simulink model "MIL4L3_SW6_V1_20220211"  (R2018b)
settings: Solver=FixedStepAuto  StartTime=0.0  StopTime=inf  FixedStep=0.001  RelTol=1e-3
PreLoadFcn:
  | A0_MILtest;
undefined symbols (not defined in the file or in its folder): Clb_ICADirect_LaneDisp_StateFive, Clb_ICADirect_LaneDisp_StateFour, Clb_ICADirect_LaneDisp_StateOne, Clb_ICADirect_LaneDisp_StateThree, Clb_ICADirect_LaneDisp_StateTwo, Clb_ICADirect_LaneDisp_StateZero, Clb_ICADirect_LaneDispSW, Clb_ICADirect_TrnLghtsCom_Switch, Clb_ICADirect_TrnLghtsCom_Value, Clb_ICADirect_TrnLghtsCrtl_Inhb, IMAP_Clb_ACU_Driver_Belt, IMAP_Clb_ACU_Driver_Belt_Over, IMAP_Clb_ACU_Passenger_Belt, IMAP_Clb_ACU_Passenger_Belt_Over, IMAP_Clb_ACU_RearLeft_Belt, IMAP_Clb_ACU_RearLeft_Belt_Over, IMAP_Clb_ACU_RearMiddle_Belt, IMAP_Clb_ACU_RearMiddle_Belt_Over, IMAP_Clb_ACU_RearRight_Belt, IMAP_Clb_ACU_RearRight_Belt_Over, IMAP_Clb_AEB_Switch, IMAP_Clb_AEB_Switch_Over, IMAP_Clb_ALC_TLC_Mode, IMAP_Clb_ALC_TLC_Mode_Over, IMAP_Clb_BCM_Battery_Voltage, IMAP_Clb_BCM_Battery_Voltage_Over, IMAP_Clb_BCM_BrakeLamp_State, IMAP_Clb_BCM_BrakeLamp_State_Over, IMAP_Clb_BCM_CHMSL_Status, IMAP_Clb_BCM_CHMSL_Status_Over, IMAP_Clb_BCM_Door_Lock_State, IMAP_Clb_BCM_Door_Lock_State_Over, IMAP_Clb_BCM_FrontWiper_State, IMAP_Clb_BCM_FrontWiper_State_Over, IMAP_Clb_BCM_FrontWiper_Switch, IMAP_Clb_BCM_FrontWiper_Switch_Over, IMAP_Clb_BCM_HazardLamp, IMAP_Clb_BCM_HazardLamp_Over, IMAP_Clb_BCM_HazardLamp_Switch, IMAP_Clb_BCM_HazardLamp_Switch_Over, IMAP_Clb_BCM_HighBeam_State, IMAP_Clb_BCM_HighBeam_State_Over, IMAP_Clb_BCM_Ignition_State, IMAP_Clb_BCM_Ignition_State_Over, IMAP_Clb_BCM_IHBC_Enabled, IMAP_Clb_BCM_IHBC_Enabled_Over, IMAP_Clb_BCM_Left_Light, IMAP_Clb_BCM_Left_Light_Over, IMAP_Clb_BCM_LeftTurn_Switch, IMAP_Clb_BCM_LeftTurn_Switch_Over, IMAP_Clb_BCM_LF_Door_State, IMAP_Clb_BCM_LF_Door_State_Over, IMAP_Clb_BCM_LowBeam_State, IMAP_Clb_BCM_LowBeam_State_Over, IMAP_Clb_BCM_LR_Door_State, IMAP_Clb_BCM_LR_Door_State_Over, IMAP_Clb_BCM_RF_Door_State, IMAP_Clb_BCM_RF_Door_State_Over, IMAP_Clb_BCM_Right_Light, IMAP_Clb_BCM_Right_Light_Over ... (+547)
libraries: CarMaker4SL x2153, simulink x292, dspstat3 x3, canmsglib x2, simulink_extras x1
(part 50 of 52)

== system MIL4L3_SW6_V1_20220211/CarMaker/VehicleControl/OMAP/OMAP1/Runnable_OMAP_10ms_sys/OMAP_Module/ICA_Direct_G59/ICA_Define/Subsystem1/Dspl/DsplPrcs/Txt/TxtFromACC ==
  note: 有没有收到方向盘限幅的影响
  note: 用于放弃变道的接管预留
  TxtFromACC_stTHState : Inport
  TxtFromACC_stLstTHState : Inport  Port=2
  TxtFromACC_stACCTxtDspl : Inport  Port=3
  TxtFromACC_stSWALimFlg : Inport  Port=4
  TxtFromACC_tiSWALimFlgDetnum : Inport  Port=5
  TxtFromACC_stTkOvStChk : Inport  Port=6
  TxtFromACC_tfAddVocCmd : Inport  Port=7
  TxtFromACC_stVehSty : Inport  Port=8
  Compare To Constant : simulink/Logic and Bit Operations/Compare To Constant  relop===  const=uint16(3)  OutDataTypeStr=boolean
  Compare To Zero : simulink/Logic and Bit Operations/Compare To Zero  relop===  OutDataTypeStr=boolean
  Constant{1,3,5,7,9,11,13,15,17,19} (10 alike) : Constant  OutDataTypeStr=uint16
  Constant{2,4,6,8,10,12,14,16,18,20} (10 alike) : Constant  Value=0  OutDataTypeStr=uint16
  Data Type Conversion14 : DataTypeConversion  OutDataTypeStr=uint16
  Data Type Conversion2 : DataTypeConversion  OutDataTypeStr=uint16
  Enabled Subsystem : Subsystem  TreatAsAtomicUnit=on
  Hold : Subsystem  TreatAsAtomicUnit=on
  If : If  NumInputs=2  IfExpression=( u1 == 3 |u1 == 4 |u1 == 6 )& u2 == 6
  If1 : If  NumInputs=2  IfExpression=( u1 == 3 |u1 == 4 |u1 == 6 )& u2 == 7
  If2 : If  NumInputs=2  IfExpression=( u1 == 3 |u1 == 4 |u1 == 6 )& u2 == 8
  If3 : If  NumInputs=3  IfExpression=u1 == 5 & u2 == 2 & u3 == 0
  If4 : If  NumInputs=2  IfExpression=u1 == 1  ElseIfExpressions=u2 == 1
  If5 : If  NumInputs=2  IfExpression=( u1 == 3 |u1 == 4 |u1 == 6 )& u2 == 12
  If6 : If  NumInputs=2  IfExpression=( u1 == 3 |u1 == 4 |u1 == 6 )& u2 == 13
  If7 : If  NumInputs=2  IfExpression=( u1 == 3 |u1 == 4 |u1 == 6 )& u2 == 14
  If8 : If  NumInputs=2  IfExpression=( u1 == 3 |u1 == 4 )& u2 == 15
  If9 : If  NumInputs=2  IfExpression=( u1 == 3 |u1 == 4 )& u2 == 16
  Logical Operator : Logic  Operator=OR  AllPortsSameDT=off  OutDataTypeStr=boolean
  Logical Operator1 : Logic  Inputs=3  AllPortsSameDT=off  OutDataTypeStr=boolean
  Logical Operator2 : Logic  Operator=OR  AllPortsSameDT=off  OutDataTypeStr=boolean
  Merge{,1..3,5..9} (9 alike) : Merge
  Merge4 : Merge  Inputs=3
  RdrBlkInhib : Subsystem
  Start : Subsystem  TreatAsAtomicUnit=on
  Start1 : Subsystem  TreatAsAtomicUnit=on
  Start2 : Subsystem  TreatAsAtomicUnit=on
  Start3 : Subsystem  TreatAsAtomicUnit=on
  Start4 : Subsystem  TreatAsAtomicUnit=on
  Start5 : Subsystem  TreatAsAtomicUnit=on
  Start6 : Subsystem  TreatAsAtomicUnit=on
  Start7 : Subsystem  TreatAsAtomicUnit=on
  Start8 : Subsystem  TreatAsAtomicUnit=on
  Start9 : Subsystem  TreatAsAtomicUnit=on
  Stop : Subsystem  TreatAsAtomicUnit=on
  Stop1 : Subsystem  TreatAsAtomicUnit=on
  Stop2 : Subsystem  TreatAsAtomicUnit=on
  Stop3 : Subsystem  TreatAsAtomicUnit=on
  Stop4 : Subsystem  TreatAsAtomicUnit=on
  Stop5 : Subsystem  TreatAsAtomicUnit=on
  Stop6 : Subsystem  TreatAsAtomicUnit=on
  Stop7 : Subsystem  TreatAsAtomicUnit=on
  Stop8 : Subsystem  TreatAsAtomicUnit=on
  Stop9 : Subsystem  TreatAsAtomicUnit=on
  Unit Delay1 : UnitDelay  SampleTime=-1
  TxtFromACC_stGoReq : Outport
  TxtFromACC_stTkOv : Outport  Port=2
  TxtFromACC_stImmdTkOv : Outport  Port=3
  TxtFromACC_stRdrBlk : Outport  Port=4
  TxtFromACC_stPressSet : Outport  Port=5
  TxtFromACC_stResEPB : Outport  Port=6
  TxtFromACC_stResBrkPedal : Outport  Port=7
  TxtFromACC_stISAToOn : Outport  Port=8
  TxtFromACC_stISAToOff : Outport  Port=9
  wires:
  Stop/1(Out1) -> Merge/2
  Constant2/1 -> Stop/1(In1)
  If/1 -> Start/Action
  Constant1/1 -> Start/1(In1)
  Start/1(Out1) -> Merge/1
  Merge/1 -> TxtFromACC_stGoReq/1
  If/2 -> Stop/Action
  TxtFromACC_stTHState/1 -> [THState]
  If1/2 -> Stop1/Action
  Stop1/1(Out1) -> Merge1/2
  Start1/1(Out1) -> Merge1/1
  Constant4/1 -> Stop1/1(In1)
  If1/1 -> Start1/Action
  Merge1/1 -> TxtFromACC_stTkOv/1
  Constant3/1 -> Start1/1(In1)
  If2/2 -> Stop2/Action
  Stop2/1(Out1) -> Merge2/2
  Start2/1(Out1) -> Merge2/1
  Constant6/1 -> Stop2/1(In1)
  If2/1 -> Start2/Action
  Constant5/1 -> Start2/1(In1)
  TxtFromACC_stLstTHState/1 -> RdrBlkInhib/2(RdrBlkInhib_stLstTHState)
  TxtFromACC_stACCTxtDspl/1 -> [ACCTxtDspl]
  [THState] -> If/1
  [ACCTxtDspl] -> If/2
  [THState] -> If1/1
  [ACCTxtDspl] -> If1/2
  [THState] -> If2/1
  [ACCTxtDspl] -> If2/2
  [THState] -> RdrBlkInhib/1(RdrBlkInhib_stTHState)
  [ACCTxtDspl] -> RdrBlkInhib/3(RdrBlkInhib_stACCTxtDspl)
  If3/2 -> Stop3/Action
  Start3/1(Out1) -> Merge3/1
  If3/1 -> Start3/Action
  Constant7/1 -> Start3/1(In1)
  Constant8/1 -> Stop3/1(In1)
  Stop3/1(Out1) -> Merge3/2
  [ACCTxtDspl] -> If3/2
  [THState] -> If3/1
  Merge3/1 -> TxtFromACC_stRdrBlk/1
  RdrBlkInhib/1(RdrBlkInhib_stRdrBlkInhibFlg) -> If3/3
  TxtFromACC_stSWALimFlg/1 -> Logical Operator1/3
  TxtFromACC_stTkOvStChk/1 -> If4/2
  If4/2 -> Stop4/Action
  Stop4/1(Out1) -> Merge4/2
  Start4/1(Out1) -> Merge4/1
  Constant10/1 -> Stop4/1(In1)
  If4/1 -> Start4/Action
  Constant9/1 -> Start4/1(In1)
  Hold/1(Out1) -> Merge4/3
  Unit Delay1/1 -> Hold/1(In1)
  Merge4/1 -> Logical Operator/2, Unit Delay1/1
  If4/3 -> Hold/Action
  Merge2/1 -> Logical Operator/1
  Logical Operator/1 -> Data Type Conversion14/1
  Data Type Conversion14/1 -> TxtFromACC_stImmdTkOv/1
  [THState] -> Compare To Constant/1
  Compare To Constant/1 -> Logical Operator1/2
  Data Type Conversion2/1 -> If4/1
  TxtFromACC_tiSWALimFlgDetnum/1 -> Enabled Subsystem/1(Num)
  Enabled Subsystem/1(Triger) -> Logical Operator2/1
  Logical Operator1/1 -> Enabled Subsystem/Enable
  [ACCTxtDspl] -> If5/2
  [THState] -> If5/1
  If5/2 -> Stop5/Action
  Merge5/1 -> TxtFromACC_stPressSet/1
  Start5/1(Out1) -> Merge5/1
  Constant11/1 -> Start5/1(In1)
  If5/1 -> Start5/Action
  Constant12/1 -> Stop5/1(In1)
  Stop5/1(Out1) -> Merge5/2
  Stop6/1(Out1) -> Merge6/2
  Constant14/1 -> Stop6/1(In1)
  If6/1 -> Start6/Action
  Constant13/1 -> Start6/1(In1)
  Start6/1(Out1) -> Merge6/1
  Merge6/1 -> TxtFromACC_stResEPB/1
  If6/2 -> Stop6/Action
  [THState] -> If6/1
  [ACCTxtDspl] -> If6/2
  [ACCTxtDspl] -> If7/2
  [THState] -> If7/1
  If7/2 -> Stop7/Action
  Merge7/1 -> TxtFromACC_stResBrkPedal/1
  Start7/1(Out1) -> Merge7/1
  Constant15/1 -> Start7/1(In1)
  If7/1 -> Start7/Action
  Constant16/1 -> Stop7/1(In1)
  Stop7/1(Out1) -> Merge7/2
  Stop8/1(Out1) -> Merge8/2
  Constant18/1 -> Stop8/1(In1)
  If8/1 -> Start8/Action
  Constant17/1 -> Start8/1(In1)
  Start8/1(Out1) -> Merge8/1
  Merge8/1 -> TxtFromACC_stISAToOn/1
  If8/2 -> Stop8/Action
  [THState] -> If8/1
  [ACCTxtDspl] -> If8/2
  [ACCTxtDspl] -> If9/2
  [THState] -> If9/1
  If9/2 -> Stop9/Action
  Merge9/1 -> TxtFromACC_stISAToOff/1
  Start9/1(Out1) -> Merge9/1
  Constant19/1 -> Start9/1(In1)
  If9/1 -> Start9/Action
  Constant20/1 -> Stop9/1(In1)
  Stop9/1(Out1) -> Merge9/2
  TxtFromACC_tfAddVocCmd/1 -> Logical Operator2/2
  Logical Operator2/1 -> Data Type Conversion2/1
  Compare To Zero/1 -> Logical Operator1/1
  TxtFromACC_stVehSty/1 -> Compare To Zero/1

== system MIL4L3_SW6_V1_20220211/CarMaker/VehicleControl/OMAP/OMAP1/Runnable_OMAP_10ms_sys/OMAP_Module/ICA_Direct_G59/ICA_Define/Subsystem1/Dspl/DsplPrcs/Txt/TxtInactv ==
  TxtInactv_stTHState : Inport
  TxtInactv_stTHFKeyState : Inport  Port=2
  TxtInactv_stCntRst : Inport  Port=3
  Constant1 : Constant  OutDataTypeStr=uint16
  Constant2 : Constant  Value=0  OutDataTypeStr=uint16
  Hold : Subsystem  TreatAsAtomicUnit=on
  If : If  NumInputs=3  IfExpression=u1 ~= 1 | u3 == 1  ElseIfExpressions=u1 == 1 & (u2 == 3 | u2 == 4)
  Merge : Merge  Inputs=3
  Start : Subsystem  TreatAsAtomicUnit=on
  Stop : Subsystem  TreatAsAtomicUnit=on
  Unit Delay1 : UnitDelay  SampleTime=-1
  TxtInactv_stInactv : Outport
  wires:
  Hold/1(Out1) -> Merge/3
  Start/1(Out1) -> Merge/2
  If/3 -> Hold/Action
  Unit Delay1/1 -> Hold/1(In1)
  If/2 -> Start/Action
  If/1 -> Stop/Action
  TxtInactv_stTHFKeyState/1 -> If/2
  Stop/1(Out1) -> Merge/1
  Merge/1 -> TxtInactv_stInactv/1, Unit Delay1/1
  TxtInactv_stTHState/1 -> If/1
  TxtInactv_stCntRst/1 -> If/3
  Constant1/1 -> Start/1(In1)
  Constant2/1 -> Stop/1(In1)

== system MIL4L3_SW6_V1_20220211/CarMaker/VehicleControl/OMAP/OMAP1/Runnable_OMAP_10ms_sys/OMAP_Module/ICA_Direct_G59/ICA_Define/Subsystem1/Dspl/DsplPrcs/Txt/TxtOff ==
  TxtOff_stTHState : Inport
  TxtOff_stLstTHState : Inport  Port=2
  Constant1 : Constant  OutDataTypeStr=uint16
  Constant2 : Constant  Value=0  OutDataTypeStr=uint16
  Hold : Subsystem  TreatAsAtomicUnit=on
  If : If  NumInputs=2  IfExpression=u1 == 0 & u2 ~= 0 & u2 ~= 5  ElseIfExpressions=u1 ~= 0
  Merge : Merge  Inputs=3
  Start : Subsystem  TreatAsAtomicUnit=on
  Stop : Subsystem  TreatAsAtomicUnit=on
  Unit Delay1 : UnitDelay  SampleTime=-1
  TxtOff_stOff : Outport
  wires:
  TxtOff_stTHState/1 -> If/1
  Merge/1 -> Unit Delay1/1, TxtOff_stOff/1
  Start/1(Out1) -> Merge/1
  TxtOff_stLstTHState/1 -> If/2
  Constant1/1 -> Start/1(In1)
  If/1 -> Start/Action
  Constant2/1 -> Stop/1(In1)
  If/2 -> Stop/Action
  Unit Delay1/1 -> Hold/1(In1)
  If/3 -> Hold/Action
  Stop/1(Out1) -> Merge/2
  Hold/1(Out1) -> Merge/3

== system MIL4L3_SW6_V1_20220211/CarMaker/VehicleControl/OMAP/OMAP1/Runnable_OMAP_10ms_sys/OMAP_Module/ICA_Direct_G59/ICA_Define/Subsystem1/Dspl/DsplPrcs/Txt/TxtOffToFault ==
  TxtOffToFault_stTHState : Inport
  TxtOffToFault_stLstTHState : Inport  Port=2
  TxtOffToFault_stACCState : Inport  Port=3
  Constant1 : Constant  OutDataTypeStr=uint16
  Constant2 : Constant  Value=0  OutDataTypeStr=uint16
  Hold : Subsystem  TreatAsAtomicUnit=on
  If : If  NumInputs=3  IfExpression=u1 == 5 & u2 == 0 & u3 ~= 15  ElseIfExpressions=u1 ~= 5 | u3 == 15
  Merge : Merge  Inputs=3
  Start : Subsystem  TreatAsAtomicUnit=on
  Stop : Subsystem  TreatAsAtomicUnit=on
  Unit Delay1 : UnitDelay  SampleTime=-1
  TxtOffToFault_stOffToFault : Outport
  wires:
  TxtOffToFault_stTHState/1 -> If/1
  Merge/1 -> Unit Delay1/1, TxtOffToFault_stOffToFault/1
  Start/1(Out1) -> Merge/1
  TxtOffToFault_stLstTHState/1 -> If/2
  TxtOffToFault_stACCState/1 -> If/3
  Constant1/1 -> Start/1(In1)
  If/1 -> Start/Action
  Constant2/1 -> Stop/1(In1)
  If/2 -> Stop/Action
  Unit Delay1/1 -> Hold/1(In1)
  If/3 -> Hold/Action
  Stop/1(Out1) -> Merge/2
  Hold/1(Out1) -> Merge/3

== system MIL4L3_SW6_V1_20220211/CarMaker/VehicleControl/OMAP/OMAP1/Runnable_OMAP_10ms_sys/OMAP_Module/ICA_Direct_G59/ICA_Define/Subsystem1/Dspl/DsplPrcs/Txt/TxtOn ==
  TxtOn_stTHState : Inport
  TxtOn_stLstTHState : Inport  Port=2
  Constant1 : Constant  OutDataTypeStr=uint16
  Constant2 : Constant  Value=0  OutDataTypeStr=uint16
  Hold : Subsystem  TreatAsAtomicUnit=on
  If : If  NumInputs=2  IfExpression=u1 == 8 & u2 == 0  ElseIfExpressions=u1 == 0 | u1 == 5
  Merge : Merge  Inputs=3
  Start : Subsystem  TreatAsAtomicUnit=on
  Stop : Subsystem  TreatAsAtomicUnit=on
  Unit Delay1 : UnitDelay  SampleTime=-1
  TxtOn_stOn : Outport
  wires:
  TxtOn_stTHState/1 -> If/1
  Merge/1 -> Unit Delay1/1, TxtOn_stOn/1
  Start/1(Out1) -> Merge/1
  TxtOn_stLstTHState/1 -> If/2
  Constant1/1 -> Start/1(In1)
  If/1 -> Start/Action
  Constant2/1 -> Stop/1(In1)
  If/2 -> Stop/Action
  Unit Delay1/1 -> Hold/1(In1)
  If/3 -> Hold/Action
  Stop/1(Out1) -> Merge/2
  Hold/1(Out1) -> Merge/3

== system MIL4L3_SW6_V1_20220211/CarMaker/VehicleControl/OMAP/OMAP1/Runnable_OMAP_10ms_sys/OMAP_Module/ICA_Direct_G59/ICA_Define/Subsystem1/Dspl/DsplPrcs/Txt/TxtOnToFault ==
  TxtOnToFault_stTHState : Inport
  TxtOnToFault_stLstTHState : Inport  Port=2
  Constant1 : Constant  OutDataTypeStr=uint16
  Constant2 : Constant  Value=0  OutDataTypeStr=uint16
  Hold : Subsystem  TreatAsAtomicUnit=on
  If : If  NumInputs=2  IfExpression=u1 == 5 & u2 ~= 0 & u2 ~= 5  ElseIfExpressions=u1 ~= 5
  Merge : Merge  Inputs=3
  Start : Subsystem  TreatAsAtomicUnit=on
  Stop : Subsystem  TreatAsAtomicUnit=on
  Unit Delay1 : UnitDelay  SampleTime=-1
  TxtOnToFault_stOnToFault : Outport
  wires:
  Hold/1(Out1) -> Merge/3
  Stop/1(Out1) -> Merge/2
  If/3 -> Hold/Action
  Unit Delay1/1 -> Hold/1(In1)
  If/2 -> Stop/Action
  Constant2/1 -> Stop/1(In1)
  If/1 -> Start/Action
  Constant1/1 -> Start/1(In1)
  TxtOnToFault_stLstTHState/1 -> If/2
  Start/1(Out1) -> Merge/1
  Merge/1 -> TxtOnToFault_stOnToFault/1, Unit Delay1/1
  TxtOnToFault_stTHState/1 -> If/1

== system MIL4L3_SW6_V1_20220211/CarMaker/VehicleControl/OMAP/OMAP1/Runnable_OMAP_10ms_sys/OMAP_Module/ICA_Direct_G59/ICA_Define/Subsystem1/Dspl/DsplPrcs/Txt/Txt_Tlimit ==
  incrcondition : Inport
  maxlimit : Inport  Port=2
  Compare To Constant : simulink/Logic and Bit Operations/Compare To Constant  relop===  const=boolean(1)  OutDataTypeStr=boolean
  Compare To Constant1 : simulink/Logic and Bit Operations/Compare To Constant  relop===  const=uint16(0)  OutDataTypeStr=boolean
  Constant : Constant  Value=0  OutDataTypeStr=uint16
  Constant1 : Constant  Value=0  OutDataTypeStr=uint16
  Constant2 : Constant  OutDataTypeStr=uint16
  Constant4 : Constant  OutDataTypeStr=uint16
  Constant5 : Constant  Value=0  OutDataTypeStr=uint16
  Data Type Conversion3 : DataTypeConversion  OutDataTypeStr=uint16
  Detect Fall Nonpositive : simulink/Logic and Bit Operations/Detect Fall Nonpositive  vinit=0  OutDataTypeStr=boolean
      settings: SourceProductName=Simulink  SourceProductBaseCode=SL
  Detect Rise Positive : simulink/Logic and Bit Operations/Detect Rise Positive  vinit=0  OutDataTypeStr=boolean
  Hold : Subsystem  TreatAsAtomicUnit=on
  If : If  NumInputs=3  IfExpression=u1 == 1  ElseIfExpressions=u2 == 1 | u3 == 1
  Logical Operator : Logic  Operator=OR  AllPortsSameDT=off  OutDataTypeStr=boolean
  Merge : Merge  Inputs=3
  MinMax1 : MinMax  Inputs=2  OutDataTypeStr=uint16  InputSameDT=on
  Relational Operator : RelationalOperator  Operator=<=  OutDataTypeStr=boolean  RndMeth=Nearest
  Start : Subsystem  TreatAsAtomicUnit=on
  Stop : Subsystem  TreatAsAtomicUnit=on
  Sum : Sum  OutDataTypeStr=Inherit: Inherit via back propagation  InputSameDT=on
  Unit Delay : UnitDelay  SampleTime=-1
  Unit Delay1 : UnitDelay  SampleTime=-1
  Unit Delay3 : UnitDelay  SampleTime=-1
  inc switch : Switch  Criteria=u2 ~= 0  Threshold=1  OutDataTypeStr=Inherit: Inherit via back propagation  InputSameDT=on
  reset switch : Switch  Criteria=u2 ~= 0  Threshold=1  OutDataTypeStr=Inherit: Inherit via back propagation  InputSameDT=on
  counter_status : Outport
  counter_reset : Outport  Port=2
  wires:
  Unit Delay/1 -> Sum/2
  maxlimit/1 -> Relational Operator/1, MinMax1/2
  MinMax1/1 -> reset switch/3
  Hold/1(Out1) -> Merge/3
  Unit Delay1/1 -> Hold/1(In1)
  If/3 -> Hold/Action
  Stop/1(Out1) -> Merge/2
  Constant4/1 -> Start/1(In1)
  If/1 -> Start/Action
  Start/1(Out1) -> Merge/1
  If/2 -> Stop/Action
  Constant5/1 -> Stop/1(In1)
  incrcondition/1 -> Detect Rise Positive/1, Detect Fall Nonpositive/1
  Detect Rise Positive/1 -> If/1
  Detect Fall Nonpositive/1 -> If/2
  Sum/1 -> MinMax1/1
  reset switch/1 -> Relational Operator/2, Unit Delay/1
  Constant1/1 -> reset switch/1
  Relational Operator/1 -> Unit Delay3/1
  [reset] -> If/3
  [reset] -> Compare To Constant/1
  Constant2/1 -> inc switch/1
  Constant/1 -> inc switch/3
  inc switch/1 -> Sum/1
  Logical Operator/1 -> reset switch/2
  Data Type Conversion3/1 -> counter_reset/1
  Unit Delay3/1 -> Data Type Conversion3/1, [reset]
  Compare To Constant/1 -> Logical Operator/2
  Merge/1 -> Compare To Constant1/1, counter_status/1, inc switch/2, Unit Delay1/1
  Compare To Constant1/1 -> Logical Operator/1

== system MIL4L3_SW6_V1_20220211/CarMaker/VehicleControl/OMAP/OMAP1/Runnable_OMAP_10ms_sys/OMAP_Module/ICA_Direct_G59/ICA_Define/Subsystem1/Dspl/DsplPrcs/Txt/Txt_Tlimit1 ==
  incrcondition : Inport
  maxlimit : Inport  Port=2
  Compare To Constant : simulink/Logic and Bit Operations/Compare To Constant  relop===  const=boolean(1)  OutDataTypeStr=boolean
  Compare To Constant1 : simulink/Logic and Bit Operations/Compare To Constant  relop===  const=uint16(0)  OutDataTypeStr=boolean
  Constant : Constant  Value=0  OutDataTypeStr=uint16
  Constant1 : Constant  Value=0  OutDataTypeStr=uint16
  Constant2 : Constant  OutDataTypeStr=uint16
  Constant4 : Constant  OutDataTypeStr=uint16
  Constant5 : Constant  Value=0  OutDataTypeStr=uint16
  Data Type Conversion3 : DataTypeConversion  OutDataTypeStr=uint16
  Detect Fall Nonpositive : simulink/Logic and Bit Operations/Detect Fall Nonpositive  vinit=0  OutDataTypeStr=boolean
      settings: SourceProductName=Simulink  SourceProductBaseCode=SL
  Detect Rise Positive : simulink/Logic and Bit Operations/Detect Rise Positive  vinit=0  OutDataTypeStr=boolean
  Hold : Subsystem  TreatAsAtomicUnit=on
  If : If  NumInputs=3  IfExpression=u1 == 1  ElseIfExpressions=u2 == 1 | u3 == 1
  Logical Operator : Logic  Operator=OR  AllPortsSameDT=off  OutDataTypeStr=boolean
  Merge : Merge  Inputs=3
  MinMax1 : MinMax  Inputs=2  OutDataTypeStr=uint16  InputSameDT=on
  Relational Operator : RelationalOperator  Operator=<=  OutDataTypeStr=boolean  RndMeth=Nearest
  Start : Subsystem  TreatAsAtomicUnit=on
  Stop : Subsystem  TreatAsAtomicUnit=on
  Sum : Sum  OutDataTypeStr=Inherit: Inherit via back propagation  InputSameDT=on
  Unit Delay : UnitDelay  SampleTime=-1
  Unit Delay1 : UnitDelay  SampleTime=-1
  Unit Delay3 : UnitDelay  SampleTime=-1
  inc switch : Switch  Criteria=u2 ~= 0  Threshold=1  OutDataTypeStr=Inherit: Inherit via back propagation  InputSameDT=on
  reset switch : Switch  Criteria=u2 ~= 0  Threshold=1  OutDataTypeStr=Inherit: Inherit via back propagation  InputSameDT=on
  counter_status : Outport
  counter_reset : Outport  Port=2
  wires:
  Compare To Constant1/1 -> Logical Operator/1
  Merge/1 -> Unit Delay1/1, inc switch/2, counter_status/1, Compare To Constant1/1
  Compare To Constant/1 -> Logical Operator/2
  Unit Delay3/1 -> [reset], Data Type Conversion3/1
  Data Type Conversion3/1 -> counter_reset/1
  Logical Operator/1 -> reset switch/2
  inc switch/1 -> Sum/1
  Constant/1 -> inc switch/3
  Constant2/1 -> inc switch/1
  [reset] -> Compare To Constant/1
  [reset] -> If/3
  Relational Operator/1 -> Unit Delay3/1
  Constant1/1 -> reset switch/1
  reset switch/1 -> Unit Delay/1, Relational Operator/2
  Sum/1 -> MinMax1/1
  Detect Fall Nonpositive/1 -> If/2
  Detect Rise Positive/1 -> If/1
  incrcondition/1 -> Detect Fall Nonpositive/1, Detect Rise Positive/1
  Constant5/1 -> Stop/1(In1)
  If/2 -> Stop/Action
  Start/1(Out1) -> Merge/1
  If/1 -> Start/Action
  Constant4/1 -> Start/1(In1)
  Stop/1(Out1) -> Merge/2
  If/3 -> Hold/Action
  Unit Delay1/1 -> Hold/1(In1)
  Hold/1(Out1) -> Merge/3
  MinMax1/1 -> reset switch/3
  maxlimit/1 -> MinMax1/2, Relational Operator/1
  Unit Delay/1 -> Sum/2

== system MIL4L3_SW6_V1_20220211/CarMaker/VehicleControl/OMAP/OMAP1/Runnable_OMAP_10ms_sys/OMAP_Module/ICA_Direct_G59/ICA_Define/Subsystem1/Dspl/DsplPrcs/Txt/Txt_Tlimit2 ==
  incrcondition : Inport
  maxlimit : Inport  Port=2
  Compare To Constant : simulink/Logic and Bit Operations/Compare To Constant  relop===  const=boolean(1)  OutDataTypeStr=boolean
  Compare To Constant1 : simulink/Logic and Bit Operations/Compare To Constant  relop===  const=uint16(0)  OutDataTypeStr=boolean
  Constant : Constant  Value=0  OutDataTypeStr=uint16
  Constant1 : Constant  Value=0  OutDataTypeStr=uint16
  Constant2 : Constant  OutDataTypeStr=uint16
  Constant4 : Constant  OutDataTypeStr=uint16
  Constant5 : Constant  Value=0  OutDataTypeStr=uint16
  Data Type Conversion3 : DataTypeConversion  OutDataTypeStr=uint16
  Detect Fall Nonpositive : simulink/Logic and Bit Operations/Detect Fall Nonpositive  vinit=0  OutDataTypeStr=boolean
      settings: SourceProductName=Simulink  SourceProductBaseCode=SL
  Detect Rise Positive : simulink/Logic and Bit Operations/Detect Rise Positive  vinit=0  OutDataTypeStr=boolean
  Hold : Subsystem  TreatAsAtomicUnit=on
  If : If  NumInputs=3  IfExpression=u1 == 1  ElseIfExpressions=u2 == 1 | u3 == 1
  Logical Operator : Logic  Operator=OR  AllPortsSameDT=off  OutDataTypeStr=boolean
  Merge : Merge  Inputs=3
  MinMax1 : MinMax  Inputs=2  OutDataTypeStr=uint16  InputSameDT=on
  Relational Operator : RelationalOperator  Operator=<=  OutDataTypeStr=boolean  RndMeth=Nearest
  Start : Subsystem  TreatAsAtomicUnit=on
  Stop : Subsystem  TreatAsAtomicUnit=on
  Sum : Sum  OutDataTypeStr=Inherit: Inherit via back propagation  InputSameDT=on
  Unit Delay : UnitDelay  SampleTime=-1
  Unit Delay1 : UnitDelay  SampleTime=-1
  Unit Delay3 : UnitDelay  SampleTime=-1
  inc switch : Switch  Criteria=u2 ~= 0  Threshold=1  OutDataTypeStr=Inherit: Inherit via back propagation  InputSameDT=on
  reset switch : Switch  Criteria=u2 ~= 0  Threshold=1  OutDataTypeStr=Inherit: Inherit via back propagation  InputSameDT=on
  counter_status : Outport
  counter_reset : Outport  Port=2
  wires:
  Unit Delay/1 -> Sum/2
  maxlimit/1 -> Relational Operator/1, MinMax1/2
  MinMax1/1 -> reset switch/3
  Hold/1(Out1) -> Merge/3
  Unit Delay1/1 -> Hold/1(In1)
  If/3 -> Hold/Action
  Stop/1(Out1) -> Merge/2
  Constant4/1 -> Start/1(In1)
  If/1 -> Start/Action
  Start/1(Out1) -> Merge/1
  If/2 -> Stop/Action
  Constant5/1 -> Stop/1(In1)
  incrcondition/1 -> Detect Rise Positive/1, Detect Fall Nonpositive/1
  Detect Rise Positive/1 -> If/1
  Detect Fall Nonpositive/1 -> If/2
  Sum/1 -> MinMax1/1
  reset switch/1 -> Relational Operator/2, Unit Delay/1
  Constant1/1 -> reset switch/1
  Relational Operator/1 -> Unit Delay3/1
  [reset] -> If/3
  [reset] -> Compare To Constant/1
  Constant2/1 -> inc switch/1
  Constant/1 -> inc switch/3
  inc switch/1 -> Sum/1
  Logical Operator/1 -> reset switch/2
  Data Type Conversion3/1 -> counter_reset/1
  Unit Delay3/1 -> Data Type Conversion3/1, [reset]
  Compare To Constant/1 -> Logical Operator/2
  Merge/1 -> Compare To Constant1/1, counter_status/1, inc switch/2, Unit Delay1/1
  Compare To Constant1/1 -> Logical Operator/1

== system MIL4L3_SW6_V1_20220211/CarMaker/VehicleControl/OMAP/OMAP1/Runnable_OMAP_10ms_sys/OMAP_Module/ICA_Direct_G59/ICA_Define/Subsystem1/Dspl/DsplPrcs/Txt/Txt_Tlimit3 ==
  incrcondition : Inport
  maxlimit : Inport  Port=2
  Compare To Constant : simulink/Logic and Bit Operations/Compare To Constant  relop===  const=boolean(1)  OutDataTypeStr=boolean
  Compare To Constant1 : simulink/Logic and Bit Operations/Compare To Constant  relop===  const=uint16(0)  OutDataTypeStr=boolean
  Constant : Constant  Value=0  OutDataTypeStr=uint16
  Constant1 : Constant  Value=0  OutDataTypeStr=uint16
  Constant2 : Constant  OutDataTypeStr=uint16
  Constant4 : Constant  OutDataTypeStr=uint16
  Constant5 : Constant  Value=0  OutDataTypeStr=uint16
  Data Type Conversion3 : DataTypeConversion  OutDataTypeStr=uint16
  Detect Fall Nonpositive : simulink/Logic and Bit Operations/Detect Fall Nonpositive  vinit=0  OutDataTypeStr=boolean
      settings: SourceProductName=Simulink  SourceProductBaseCode=SL
  Detect Rise Positive : simulink/Logic and Bit Operations/Detect Rise Positive  vinit=0  OutDataTypeStr=boolean
  Hold : Subsystem  TreatAsAtomicUnit=on
  If : If  NumInputs=3  IfExpression=u1 == 1  ElseIfExpressions=u2 == 1 | u3 == 1
  Logical Operator : Logic  Operator=OR  AllPortsSameDT=off  OutDataTypeStr=boolean
  Merge : Merge  Inputs=3
  MinMax1 : MinMax  Inputs=2  OutDataTypeStr=uint16  InputSameDT=on
  Relational Operator : RelationalOperator  Operator=<=  OutDataTypeStr=boolean  RndMeth=Nearest
  Start : Subsystem  TreatAsAtomicUnit=on
  Stop : Subsystem  TreatAsAtomicUnit=on
  Sum : Sum  OutDataTypeStr=Inherit: Inherit via back propagation  InputSameDT=on
  Unit Delay : UnitDelay  SampleTime=-1
  Unit Delay1 : UnitDelay  SampleTime=-1
  Unit Delay3 : UnitDelay  SampleTime=-1
  inc switch : Switch  Criteria=u2 ~= 0  Threshold=1  OutDataTypeStr=Inherit: Inherit via back propagation  InputSameDT=on
  reset switch : Switch  Criteria=u2 ~= 0  Threshold=1  OutDataTypeStr=Inherit: Inherit via back propagation  InputSameDT=on
  counter_status : Outport
  counter_reset : Outport  Port=2
  wires:
  Compare To Constant1/1 -> Logical Operator/1
  Merge/1 -> Unit Delay1/1, inc switch/2, counter_status/1, Compare To Constant1/1
  Compare To Constant/1 -> Logical Operator/2
  Unit Delay3/1 -> [reset], Data Type Conversion3/1
  Data Type Conversion3/1 -> counter_reset/1
  Logical Operator/1 -> reset switch/2
  inc switch/1 -> Sum/1
  Constant/1 -> inc switch/3
  Constant2/1 -> inc switch/1
  [reset] -> Compare To Constant/1
  [reset] -> If/3
  Relational Operator/1 -> Unit Delay3/1
  Constant1/1 -> reset switch/1
  reset switch/1 -> Unit Delay/1, Relational Operator/2
  Sum/1 -> MinMax1/1
  Detect Fall Nonpositive/1 -> If/2
  Detect Rise Positive/1 -> If/1
  incrcondition/1 -> Detect Fall Nonpositive/1, Detect Rise Positive/1
  Constant5/1 -> Stop/1(In1)
  If/2 -> Stop/Action
  Start/1(Out1) -> Merge/1
  If/1 -> Start/Action
  Constant4/1 -> Start/1(In1)
  Stop/1(Out1) -> Merge/2
  If/3 -> Hold/Action
  Unit Delay1/1 -> Hold/1(In1)
  Hold/1(Out1) -> Merge/3
  MinMax1/1 -> reset switch/3
  maxlimit/1 -> MinMax1/2, Relational Operator/1
  Unit Delay/1 -> Sum/2

== system MIL4L3_SW6_V1_20220211/CarMaker/VehicleControl/OMAP/OMAP1/Runnable_OMAP_10ms_sys/OMAP_Module/ICA_Direct_G59/ICA_Define/Subsystem1/Dspl/DsplPrcs/Txt/Txt_Tlimit4 ==
  incrcondition : Inport
  maxlimit : Inport  Port=2
  Compare To Constant : simulink/Logic and Bit Operations/Compare To Constant  relop===  const=boolean(1)  OutDataTypeStr=boolean
  Compare To Constant1 : simulink/Logic and Bit Operations/Compare To Constant  relop===  const=uint16(0)  OutDataTypeStr=boolean
  Constant : Constant  Value=0  OutDataTypeStr=uint16
  Constant1 : Constant  Value=0  OutDataTypeStr=uint16
  Constant2 : Constant  OutDataTypeStr=uint16
  Constant4 : Constant  OutDataTypeStr=uint16
  Constant5 : Constant  Value=0  OutDataTypeStr=uint16
  Data Type Conversion3 : DataTypeConversion  OutDataTypeStr=uint16
  Detect Fall Nonpositive : simulink/Logic and Bit Operations/Detect Fall Nonpositive  vinit=0  OutDataTypeStr=boolean
      settings: SourceProductName=Simulink  SourceProductBaseCode=SL
  Detect Rise Positive : simulink/Logic and Bit Operations/Detect Rise Positive  vinit=0  OutDataTypeStr=boolean
  Hold : Subsystem  TreatAsAtomicUnit=on
  If : If  NumInputs=3  IfExpression=u1 == 1  ElseIfExpressions=u2 == 1 | u3 == 1
  Logical Operator : Logic  Operator=OR  AllPortsSameDT=off  OutDataTypeStr=boolean
  Merge : Merge  Inputs=3
  MinMax1 : MinMax  Inputs=2  OutDataTypeStr=uint16  InputSameDT=on
  Relational Operator : RelationalOperator  Operator=<=  OutDataTypeStr=boolean  RndMeth=Nearest
  Start : Subsystem  TreatAsAtomicUnit=on
  Stop : Subsystem  TreatAsAtomicUnit=on
  Sum : Sum  OutDataTypeStr=Inherit: Inherit via back propagation  InputSameDT=on
  Unit Delay : UnitDelay  SampleTime=-1
  Unit Delay1 : UnitDelay  SampleTime=-1
  Unit Delay3 : UnitDelay  SampleTime=-1
  inc switch : Switch  Criteria=u2 ~= 0  Threshold=1  OutDataTypeStr=Inherit: Inherit via back propagation  InputSameDT=on
  reset switch : Switch  Criteria=u2 ~= 0  Threshold=1  OutDataTypeStr=Inherit: Inherit via back propagation  InputSameDT=on
  counter_status : Outport
  counter_reset : Outport  Port=2
  wires:
  Unit Delay/1 -> Sum/2
  maxlimit/1 -> Relational Operator/1, MinMax1/2
  MinMax1/1 -> reset switch/3
  Hold/1(Out1) -> Merge/3
  Unit Delay1/1 -> Hold/1(In1)
  If/3 -> Hold/Action
  Stop/1(Out1) -> Merge/2
  Constant4/1 -> Start/1(In1)
  If/1 -> Start/Action
  Start/1(Out1) -> Merge/1
  If/2 -> Stop/Action
  Constant5/1 -> Stop/1(In1)
  incrcondition/1 -> Detect Rise Positive/1, Detect Fall Nonpositive/1
  Detect Rise Positive/1 -> If/1
  Detect Fall Nonpositive/1 -> If/2
  Sum/1 -> MinMax1/1
  reset switch/1 -> Relational Operator/2, Unit Delay/1
  Constant1/1 -> reset switch/1
  Relational Operator/1 -> Unit Delay3/1
  [reset] -> If/3
  [reset] -> Compare To Constant/1
  Constant2/1 -> inc switch/1
  Constant/1 -> inc switch/3
  inc switch/1 -> Sum/1
  Logical Operator/1 -> reset switch/2
  Data Type Conversion3/1 -> counter_reset/1
  Unit Delay3/1 -> Data Type Conversion3/1, [reset]
  Compare To Constant/1 -> Logical Operator/2
  Merge/1 -> Compare To Constant1/1, counter_status/1, inc switch/2, Unit Delay1/1
  Compare To Constant1/1 -> Logical Operator/1

== system MIL4L3_SW6_V1_20220211/CarMaker/VehicleControl/OMAP/OMAP1/Runnable_OMAP_10ms_sys/OMAP_Module/ICA_Direct_G59/ICA_Define/Subsystem1/Dspl/DsplPrcs/Txt/Txt_Tlimit5 ==
  incrcondition : Inport
  maxlimit : Inport  Port=2
  Compare To Constant : simulink/Logic and Bit Operations/Compare To Constant  relop===  const=boolean(1)  OutDataTypeStr=boolean
  Compare To Constant1 : simulink/Logic and Bit Operations/Compare To Constant  relop===  const=uint16(0)  OutDataTypeStr=boolean
  Constant : Constant  Value=0  OutDataTypeStr=uint16
  Constant1 : Constant  Value=0  OutDataTypeStr=uint16
  Constant2 : Constant  OutDataTypeStr=uint16
  Constant4 : Constant  OutDataTypeStr=uint16
  Constant5 : Constant  Value=0  OutDataTypeStr=uint16
  Data Type Conversion3 : DataTypeConversion  OutDataTypeStr=uint16
  Detect Fall Nonpositive : simulink/Logic and Bit Operations/Detect Fall Nonpositive  vinit=0  OutDataTypeStr=boolean
      settings: SourceProductName=Simulink  SourceProductBaseCode=SL
  Detect Rise Positive : simulink/Logic and Bit Operations/Detect Rise Positive  vinit=0  OutDataTypeStr=boolean
  Hold : Subsystem  TreatAsAtomicUnit=on
  If : If  NumInputs=3  IfExpression=u1 == 1  ElseIfExpressions=u2 == 1 | u3 == 1
  Logical Operator : Logic  Operator=OR  AllPortsSameDT=off  OutDataTypeStr=boolean
  Merge : Merge  Inputs=3
  MinMax1 : MinMax  Inputs=2  OutDataTypeStr=uint16  InputSameDT=on
  Relational Operator : RelationalOperator  Operator=<=  OutDataTypeStr=boolean  RndMeth=Nearest
  Start : Subsystem  TreatAsAtomicUnit=on
  Stop : Subsystem  TreatAsAtomicUnit=on
  Sum : Sum  OutDataTypeStr=Inherit: Inherit via back propagation  InputSameDT=on
  Unit Delay : UnitDelay  SampleTime=-1
  Unit Delay1 : UnitDelay  SampleTime=-1
  Unit Delay3 : UnitDelay  SampleTime=-1
  inc switch : Switch  Criteria=u2 ~= 0  Threshold=1  OutDataTypeStr=Inherit: Inherit via back propagation  InputSameDT=on
  reset switch : Switch  Criteria=u2 ~= 0  Threshold=1  OutDataTypeStr=Inherit: Inherit via back propagation  InputSameDT=on
  counter_status : Outport
  counter_reset : Outport  Port=2
  wires:
  Compare To Constant1/1 -> Logical Operator/1
  Merge/1 -> Unit Delay1/1, inc switch/2, counter_status/1, Compare To Constant1/1
  Compare To Constant/1 -> Logical Operator/2
  Unit Delay3/1 -> [reset], Data Type Conversion3/1
  Data Type Conversion3/1 -> counter_reset/1
  Logical Operator/1 -> reset switch/2
  inc switch/1 -> Sum/1
  Constant/1 -> inc switch/3
  Constant2/1 -> inc switch/1
  [reset] -> Compare To Constant/1
  [reset] -> If/3
  Relational Operator/1 -> Unit Delay3/1
  Constant1/1 -> reset switch/1
  reset switch/1 -> Unit Delay/1, Relational Operator/2
  Sum/1 -> MinMax1/1
  Detect Fall Nonpositive/1 -> If/2
  Detect Rise Positive/1 -> If/1
  incrcondition/1 -> Detect Fall Nonpositive/1, Detect Rise Positive/1
  Constant5/1 -> Stop/1(In1)
  If/2 -> Stop/Action
  Start/1(Out1) -> Merge/1
  If/1 -> Start/Action
  Constant4/1 -> Start/1(In1)
  Stop/1(Out1) -> Merge/2
  If/3 -> Hold/Action
  Unit Delay1/1 -> Hold/1(In1)
  Hold/1(Out1) -> Merge/3
  MinMax1/1 -> reset switch/3
  maxlimit/1 -> MinMax1/2, Relational Operator/1
  Unit Delay/1 -> Sum/2

== system MIL4L3_SW6_V1_20220211/CarMaker/VehicleControl/OMAP/OMAP1/Runnable_OMAP_10ms_sys/OMAP_Module/ICA_Direct_G59/ICA_Define/Subsystem1/Dspl/DsplPrcs/Txt/Txt_Tlimit6 ==
  incrcondition : Inport
  maxlimit : Inport  Port=2
  Compare To Constant : simulink/Logic and Bit Operations/Compare To Constant  relop===  const=boolean(1)  OutDataTypeStr=boolean
  Compare To Constant1 : simulink/Logic and Bit Operations/Compare To Constant  relop===  const=uint16(0)  OutDataTypeStr=boolean
  Constant : Constant  Value=0  OutDataTypeStr=uint16
  Constant1 : Constant  Value=0  OutDataTypeStr=uint16
  Constant2 : Constant  OutDataTypeStr=uint16
  Constant4 : Constant  OutDataTypeStr=uint16
  Constant5 : Constant  Value=0  OutDataTypeStr=uint16
  Data Type Conversion3 : DataTypeConversion  OutDataTypeStr=uint16
  Detect Fall Nonpositive : simulink/Logic and Bit Operations/Detect Fall Nonpositive  vinit=0  OutDataTypeStr=boolean
      settings: SourceProductName=Simulink  SourceProductBaseCode=SL
  Detect Rise Positive : simulink/Logic and Bit Operations/Detect Rise Positive  vinit=0  OutDataTypeStr=boolean
  Hold : Subsystem  TreatAsAtomicUnit=on
  If : If  NumInputs=3  IfExpression=u1 == 1  ElseIfExpressions=u2 == 1 | u3 == 1
  Logical Operator : Logic  Operator=OR  AllPortsSameDT=off  OutDataTypeStr=boolean
  Merge : Merge  Inputs=3
  MinMax1 : MinMax  Inputs=2  OutDataTypeStr=uint16  InputSameDT=on
  Relational Operator : RelationalOperator  Operator=<=  OutDataTypeStr=boolean  RndMeth=Nearest
  Start : Subsystem  TreatAsAtomicUnit=on
  Stop : Subsystem  TreatAsAtomicUnit=on
  Sum : Sum  OutDataTypeStr=Inherit: Inherit via back propagation  InputSameDT=on
  Unit Delay : UnitDelay  SampleTime=-1
  Unit Delay1 : UnitDelay  SampleTime=-1
  Unit Delay3 : UnitDelay  SampleTime=-1
  inc switch : Switch  Criteria=u2 ~= 0  Threshold=1  OutDataTypeStr=Inherit: Inherit via back propagation  InputSameDT=on
  reset switch : Switch  Criteria=u2 ~= 0  Threshold=1  OutDataTypeStr=Inherit: Inherit via back propagation  InputSameDT=on
  counter_status : Outport
  counter_reset : Outport  Port=2
  wires:
  Unit Delay/1 -> Sum/2
  maxlimit/1 -> Relational Operator/1, MinMax1/2
  MinMax1/1 -> reset switch/3
  Hold/1(Out1) -> Merge/3
  Unit Delay1/1 -> Hold/1(In1)
  If/3 -> Hold/Action
  Stop/1(Out1) -> Merge/2
  Constant4/1 -> Start/1(In1)
  If/1 -> Start/Action
  Start/1(Out1) -> Merge/1
  If/2 -> Stop/Action
  Constant5/1 -> Stop/1(In1)
  incrcondition/1 -> Detect Rise Positive/1, Detect Fall Nonpositive/1
  Detect Rise Positive/1 -> If/1
  Detect Fall Nonpositive/1 -> If/2
  Sum/1 -> MinMax1/1
  reset switch/1 -> Relational Operator/2, Unit Delay/1
  Constant1/1 -> reset switch/1
  Relational Operator/1 -> Unit Delay3/1
  [reset] -> If/3
  [reset] -> Compare To Constant/1
  Constant2/1 -> inc switch/1
  Constant/1 -> inc switch/3
  inc switch/1 -> Sum/1
  Logical Operator/1 -> reset switch/2
  Data Type Conversion3/1 -> counter_reset/1
  Unit Delay3/1 -> Data Type Conversion3/1, [reset]
  Compare To Constant/1 -> Logical Operator/2
  Merge/1 -> Compare To Constant1/1, counter_status/1, inc switch/2, Unit Delay1/1
  Compare To Constant1/1 -> Logical Operator/1

== system MIL4L3_SW6_V1_20220211/CarMaker/VehicleControl/OMAP/OMAP1/Runnable_OMAP_10ms_sys/OMAP_Module/ICA_Direct_G59/ICA_Define/Subsystem1/Dspl/DsplPrcs/Txt/Txt_Tlimit7 ==
  incrcondition : Inport
  maxlimit : Inport  Port=2
  Compare To Constant : simulink/Logic and Bit Operations/Compare To Constant  relop===  const=boolean(1)  OutDataTypeStr=boolean
  Compare To Constant1 : simulink/Logic and Bit Operations/Compare To Constant  relop===  const=uint16(0)  OutDataTypeStr=boolean
  Constant : Constant  Value=0  OutDataTypeStr=uint16
  Constant1 : Constant  Value=0  OutDataTypeStr=uint16
  Constant2 : Constant  OutDataTypeStr=uint16
  Constant4 : Constant  OutDataTypeStr=uint16
  Constant5 : Constant  Value=0  OutDataTypeStr=uint16
  Data Type Conversion3 : DataTypeConversion  OutDataTypeStr=uint16
  Detect Fall Nonpositive : simulink/Logic and Bit Operations/Detect Fall Nonpositive  vinit=0  OutDataTypeStr=boolean
      settings: SourceProductName=Simulink  SourceProductBaseCode=SL
  Detect Rise Positive : simulink/Logic and Bit Operations/Detect Rise Positive  vinit=0  OutDataTypeStr=boolean
  Hold : Subsystem  TreatAsAtomicUnit=on
  If : If  NumInputs=3  IfExpression=u1 == 1  ElseIfExpressions=u2 == 1 | u3 == 1
  Logical Operator : Logic  Operator=OR  AllPortsSameDT=off  OutDataTypeStr=boolean
  Merge : Merge  Inputs=3
  MinMax1 : MinMax  Inputs=2  OutDataTypeStr=uint16  InputSameDT=on
  Relational Operator : RelationalOperator  Operator=<=  OutDataTypeStr=boolean  RndMeth=Nearest
  Start : Subsystem  TreatAsAtomicUnit=on
  Stop : Subsystem  TreatAsAtomicUnit=on
  Sum : Sum  OutDataTypeStr=Inherit: Inherit via back propagation  InputSameDT=on
  Unit Delay : UnitDelay  SampleTime=-1
  Unit Delay1 : UnitDelay  SampleTime=-1
  Unit Delay3 : UnitDelay  SampleTime=-1
  inc switch : Switch  Criteria=u2 ~= 0  Threshold=1  OutDataTypeStr=Inherit: Inherit via back propagation  InputSameDT=on
  reset switch : Switch  Criteria=u2 ~= 0  Threshold=1  OutDataTypeStr=Inherit: Inherit via back propagation  InputSameDT=on
  counter_status : Outport
  counter_reset : Outport  Port=2
  wires:
  Compare To Constant1/1 -> Logical Operator/1
  Merge/1 -> Unit Delay1/1, inc switch/2, counter_status/1, Compare To Constant1/1
  Compare To Constant/1 -> Logical Operator/2
  Unit Delay3/1 -> [reset], Data Type Conversion3/1
  Data Type Conversion3/1 -> counter_reset/1
  Logical Operator/1 -> reset switch/2
  inc switch/1 -> Sum/1
  Constant/1 -> inc switch/3
  Constant2/1 -> inc switch/1
  [reset] -> Compare To Constant/1
  [reset] -> If/3
  Relational Operator/1 -> Unit Delay3/1
  Constant1/1 -> reset switch/1
  reset switch/1 -> Unit Delay/1, Relational Operator/2
  Sum/1 -> MinMax1/1
  Detect Fall Nonpositive/1 -> If/2
  Detect Rise Positive/1 -> If/1
  incrcondition/1 -> Detect Fall Nonpositive/1, Detect Rise Positive/1
  Constant5/1 -> Stop/1(In1)
  If/2 -> Stop/Action
  Start/1(Out1) -> Merge/1
  If/1 -> Start/Action
  Constant4/1 -> Start/1(In1)
  Stop/1(Out1) -> Merge/2
  If/3 -> Hold/Action
  Unit Delay1/1 -> Hold/1(In1)
  Hold/1(Out1) -> Merge/3
  MinMax1/1 -> reset switch/3
  maxlimit/1 -> MinMax1/2, Relational Operator/1
  Unit Delay/1 -> Sum/2

== system MIL4L3_SW6_V1_20220211/CarMaker/VehicleControl/OMAP/OMAP1/Runnable_OMAP_10ms_sys/OMAP_Module/ICA_Direct_G59/ICA_Define/Subsystem1/Dspl/DsplPrcs/Voc/Sum_Condition ==
  In : Inport
  Sum : Inport  Port=2
  Enable : EnablePort  StatesWhenEnabling=reset
  Add1 : Sum  OutDataTypeStr=single
  Memory : Memory  InheritSampleTime=on
  Relational Operator : RelationalOperator  OutDataTypeStr=boolean  RndMeth=Nearest
  Saturation : Saturate  UpperLimit=100000  LowerLimit=0
  Out : Outport  OutputWhenDisabled=reset  InitialOutput=0
  wires:
  Saturation/1 -> Memory/1, Relational Operator/1
  Memory/1 -> Add1/2
  Add1/1 -> Saturation/1
  In/1 -> Add1/1
  Sum/1 -> Relational Operator/2
  Relational Operator/1 -> Out/1

== system MIL4L3_SW6_V1_20220211/CarMaker/VehicleControl/Function/LKA/LKAS1/LL/LLOn/LKA/Lane Following (LF)/Trajectory Following Control (TFC)/Feedback Control (FbCtl)/Subsystem/Signal Latching2/if action  ==
  In : Inport
  Action Port : ActionPort  InitializeStates=reset  ActionType=then
  Out : Outport
  wires:
  In/1 -> Out/1

== system MIL4L3_SW6_V1_20220211/CarMaker/VehicleControl/Function/LKA/LKAS1/LL/LLOn/LKA/Plan To LaneFollowing (PTLF)/InsideJudge1/If Action Subsystem/If Action Subsystem/Signal Latching/if action  ==
  In : Inport
  Action Port : ActionPort  ActionType=then
  Out : Outport
  wires:
  In/1 -> Out/1

== system MIL4L3_SW6_V1_20220211/CarMaker/VehicleControl/Function/LKA/LKAS1/LL/LLOn/LKA/Plan To LaneFollowing (PTLF)/InsideJudge1/If Action Subsystem/If Action Subsystem/Signal Latching1/if action  ==
  In : Inport
  Action Port : ActionPort  ActionType=then
  Out : Outport
  wires:
  In/1 -> Out/1

== system MIL4L3_SW6_V1_20220211/CarMaker/VehicleControl/Function/LKA/LKAS1/LL/LLOn/LKA/Plan To LaneFollowing (PTLF)/InsideJudge1/If Action Subsystem1/If Action Subsystem/Signal Latching/if action  ==
  In : Inport
  Action Port : ActionPort  ActionType=then
  Out : Outport
  wires:
  In/1 -> Out/1

== system MIL4L3_SW6_V1_20220211/CarMaker/VehicleControl/Function/LKA/LKAS1/LL/LLOn/LKA/Plan To LaneFollowing (PTLF)/InsideJudge1/If Action Subsystem1/If Action Subsystem/Signal Latching1/if action  ==
  In : Inport
  Action Port : ActionPort  ActionType=then
  Out : Outport
  wires:
  In/1 -> Out/1

== system MIL4L3_SW6_V1_20220211/CarMaker/VehicleControl/Function/LKA/LKAS1/LL/LLOn/LL State Determination (LLStateDet)/LL State Machine Conditions (LLSMCon)/Activation Condition (ActvC)/Deviation Threshold Condition (DvtThresCon)/Deviation Threshold Judgement LDW (DvtThresJdg)/Deviation Speed Detection (DvtSpdDet)/Ph1SWA ==
  Action Port : ActionPort  InitializeStates=reset  ActionType=then
      settings: AttributesFormatString=states = %<InitializeStates>
  Constant : Constant  OutDataTypeStr=single
  Out : Outport
      settings: AttributesFormatString=%<OutputWhenDisabled> = %<InitialOutput>
  wires:
  Constant/1 -> Out/1

== system MIL4L3_SW6_V1_20220211/CarMaker/VehicleControl/Function/LKA/LKAS1/LL/LLOn/LL State Determination (LLStateDet)/LL State Machine Conditions (LLSMCon)/Activation Condition (ActvC)/Deviation Threshold Condition (DvtThresCon)/Deviation Threshold Judgement LDW (DvtThresJdg)/Deviation Speed Detection (DvtSpdDet)/Ph2SWA ==
  Action Port : ActionPort  InitializeStates=reset  ActionType=elseif
      settings: AttributesFormatString=states = %<InitializeStates>
  Constant : Constant  Value=-1  OutDataTypeStr=single
  Out : Outport
      settings: AttributesFormatString=%<OutputWhenDisabled> = %<InitialOutput>
  wires:
  Constant/1 -> Out/1

== system MIL4L3_SW6_V1_20220211/CarMaker/VehicleControl/Function/LKA/LKAS1/LL/LLOn/LL State Determination (LLStateDet)/LL State Machine Conditions (LLSMCon)/Activation Condition (ActvC)/Deviation Threshold Condition (DvtThresCon)/Deviation Threshold Judgement LDW (DvtThresJdg)/Deviation Speed Detection (DvtSpdDet)/Ph3SWA ==
  In1 : Inport
  Action Port : ActionPort  InitializeStates=reset  ActionType=else
      settings: AttributesFormatString=states = %<InitializeStates>
  Out : Outport  OutDataTypeStr=single  InitialOutput=0
      settings: AttributesFormatString=%<OutputWhenDisabled> = %<InitialOutput>
  wires:
  In1/1 -> Out/1

== system MIL4L3_SW6_V1_20220211/CarMaker/VehicleControl/Function/LKA/LKAS1/LL/LLOn/LL State Determination (LLStateDet)/LL State Machine Conditions (LLSMCon)/Activation Condition (ActvC)/Deviation Threshold Condition (DvtThresCon)/Deviation Threshold Judgement LKA (DvtThresJdg)/Deviation Speed Detection (DvtSpdDet)/Ph1SWA ==
  Action Port : ActionPort  InitializeStates=reset  ActionType=then
      settings: AttributesFormatString=states = %<InitializeStates>
  Constant : Constant  OutDataTypeStr=single
  Out : Outport
      settings: AttributesFormatString=%<OutputWhenDisabled> = %<InitialOutput>
  wires:
  Constant/1 -> Out/1

== system MIL4L3_SW6_V1_20220211/CarMaker/VehicleControl/Function/LKA/LKAS1/LL/LLOn/LL State Determination (LLStateDet)/LL State Machine Conditions (LLSMCon)/Activation Condition (ActvC)/Deviation Threshold Condition (DvtThresCon)/Deviation Threshold Judgement LKA (DvtThresJdg)/Deviation Speed Detection (DvtSpdDet)/Ph2SWA ==
  Action Port : ActionPort  InitializeStates=reset  ActionType=elseif
      settings: AttributesFormatString=states = %<InitializeStates>
  Constant : Constant  Value=-1  OutDataTypeStr=single
  Out : Outport
      settings: AttributesFormatString=%<OutputWhenDisabled> = %<InitialOutput>
  wires:
  Constant/1 -> Out/1

== system MIL4L3_SW6_V1_20220211/CarMaker/VehicleControl/Function/LKA/LKAS1/LL/LLOn/LL State Determination (LLStateDet)/LL State Machine Conditions (LLSMCon)/Activation Condition (ActvC)/Deviation Threshold Condition (DvtThresCon)/Deviation Threshold Judgement LKA (DvtThresJdg)/Deviation Speed Detection (DvtSpdDet)/Ph3SWA ==
  Action Port : ActionPort  InitializeStates=reset  ActionType=else
      settings: AttributesFormatString=states = %<InitializeStates>
  Constant : Constant  Value=0  OutDataTypeStr=single
  Out : Outport
      settings: AttributesFormatString=%<OutputWhenDisabled> = %<InitialOutput>
  wires:
  Constant/1 -> Out/1

== system MIL4L3_SW6_V1_20220211/CarMaker/VehicleControl/Function/LKA/LKAS1/LL/LLOn/LL State Determination (LLStateDet)/LL State Machine Conditions (LLSMCon)/Deactivation Condition (DeactvC)/Deviation Threshold Condition (DvtThresCon)/Deviation Threshold Judgement LDW (DvtThresJdg)/Deviation Speed Detection (DvtSpdDet)/Ph1SWA ==
  Action Port : ActionPort  InitializeStates=reset  ActionType=then
      settings: AttributesFormatString=states = %<InitializeStates>
  Constant : Constant  OutDataTypeStr=single
  Out : Outport
      settings: AttributesFormatString=%<OutputWhenDisabled> = %<InitialOutput>
  wires:
  Constant/1 -> Out/1

== system MIL4L3_SW6_V1_20220211/CarMaker/VehicleControl/Function/LKA/LKAS1/LL/LLOn/LL State Determination (LLStateDet)/LL State Machine Conditions (LLSMCon)/Deactivation Condition (DeactvC)/Deviation Threshold Condition (DvtThresCon)/Deviation Threshold Judgement LDW (DvtThresJdg)/Deviation Speed Detection (DvtSpdDet)/Ph2SWA ==
  Action Port : ActionPort  InitializeStates=reset  ActionType=elseif
      settings: AttributesFormatString=states = %<InitializeStates>
  Constant : Constant  Value=-1  OutDataTypeStr=single
  Out : Outport
      settings: AttributesFormatString=%<OutputWhenDisabled> = %<InitialOutput>
  wires:
  Constant/1 -> Out/1

== system MIL4L3_SW6_V1_20220211/CarMaker/VehicleControl/Function/LKA/LKAS1/LL/LLOn/LL State Determination (LLStateDet)/LL State Machine Conditions (LLSMCon)/Deactivation Condition (DeactvC)/Deviation Threshold Condition (DvtThresCon)/Deviation Threshold Judgement LDW (DvtThresJdg)/Deviation Speed Detection (DvtSpdDet)/Ph3SWA ==
  In1 : Inport
  Action Port : ActionPort  InitializeStates=reset  ActionType=else
      settings: AttributesFormatString=states = %<InitializeStates>
  Out : Outport  OutDataTypeStr=single  InitialOutput=0
      settings: AttributesFormatString=%<OutputWhenDisabled> = %<InitialOutput>
  wires:
  In1/1 -> Out/1

== system MIL4L3_SW6_V1_20220211/CarMaker/VehicleControl/Function/LKA/LKAS1/LL/LLOn/LL State Determination (LLStateDet)/LL State Machine Conditions (LLSMCon)/Deactivation Condition (DeactvC)/Deviation Threshold Condition (DvtThresCon)/Deviation Threshold Judgement LDW (DvtThresJdg)/Deviation Threshold Condition Synthesis (DTCSyn)/Sum Condition ==
  In : Inport
  Sum : Inport  Port=2
  Enable : EnablePort  StatesWhenEnabling=reset
      settings: AttributesFormatString=states = %<StatesWhenEnabling>
  Add1 : Sum  OutDataTypeStr=single
  Memory : Memory  InheritSampleTime=on
  Relational Operator : RelationalOperator  Operator=<=  OutDataTypeStr=boolean  RndMeth=Nearest
  Saturation : Saturate  UpperLimit=5  LowerLimit=0
      settings: AttributesFormatString="Min = %<LowerLimit>  Max = %<UpperLimit>"
  Out : Outport  OutputWhenDisabled=reset  InitialOutput=0
      settings: AttributesFormatString=%<OutputWhenDisabled> = %<InitialOutput>
  wires:
  Relational Operator/1 -> Out/1
  Memory/1 -> Add1/2
  Add1/1 -> Saturation/1
  In/1 -> Add1/1
  Sum/1 -> Relational Operator/2
  Saturation/1 -> Memory/1, Relational Operator/1

== system MIL4L3_SW6_V1_20220211/CarMaker/VehicleControl/Function/LKA/LKAS1/LL/LLOn/LL State Determination (LLStateDet)/LL State Machine Conditions (LLSMCon)/Deactivation Condition (DeactvC)/Deviation Threshold Condition (DvtThresCon)/Deviation Threshold Judgement LKA (DvtThresJdg)/Deviation Speed Detection (DvtSpdDet)/Ph1SWA ==
  Action Port : ActionPort  InitializeStates=reset  ActionType=then
      settings: AttributesFormatString=states = %<InitializeStates>
  Constant : Constant  OutDataTypeStr=single
  Out : Outport
      settings: AttributesFormatString=%<OutputWhenDisabled> = %<InitialOutput>
  wires:
  Constant/1 -> Out/1
